simulink model "DaviAraujo_FuelHeatingModel_DashBoardOK"  (R2021a)
settings: Solver=ode5  StartTime=0.0  StopTime=inf  FixedStep=0.01  RelTol=1e-3
values from neighbouring files (symbols this model uses):
  A = 0.0003*4    (= 0.0012)    [FuelHeatingModel_WS.m]
  Densidade_Combustivel = 0.774    [FuelHeatingModel_WS.m]
  EngineTemp = 90    [FuelHeatingModel_WS.m]
  Fluxo_Injetor = 2.141967    [FuelHeatingModel_WS.m]
  h = 12000    [FuelHeatingModel_WS.m]
  Lead_MaxTemp = 80    [FuelHeatingModel_WS.m]
  LeadAcid_TotalEnergy = Voltage_LeadAcid*AmpHour_LeadAcid    (= 600)    [FuelHeatingModel_WS.m]
  Lithium_MaxTemp = 80    [FuelHeatingModel_WS.m]
  Lithium_TotalEnergy = Voltage_Lithium*AmpHour_Lithium    (= 768)    [FuelHeatingModel_WS.m]
  m = (0.4*0.79)    (= 0.316)    [FuelHeatingModel_WS.m]
  Pressure_Ethanol = (P_min:((P_max-P_min)/20):P_max).^4.92    [FuelHeatingModel_WS.m]
  PWM = 0:5:100    [FuelHeatingModel_WS.m]
  RPM_Motor = 1000    [FuelHeatingModel_WS.m]
  Setpoint_ColdStart = 120    [FuelHeatingModel_WS.m]
  Setpoint_PostStart = 90    [FuelHeatingModel_WS.m]
  Temp_Ethanol = 0:6:120    [FuelHeatingModel_WS.m]
  Ts = (Ts_min:((Ts_max-Ts_min)/20):Ts_max).^0.7    [FuelHeatingModel_WS.m]
  VolumeInterno_CommonRail = 7000    [FuelHeatingModel_WS.m]
libraries: simulink x4
(part 2 of 2)

== system DaviAraujo_FuelHeatingModel_DashBoardOK/Function-Call Subsystem/Controlador de Aquecimento Pós Partida/Transient Engine ON - Fuel Heating System/Determinação do Fluxo de Combustível ==
  Fuel Density : Inport
  Fuel Pulse Width : Inport  Port=2
  Engine Speed : Inport  Port=3
  Injector Fuel Flow : Inport  Port=4
  Divide : Product  Inputs=*/
  Duração do Ciclo (ms) : Product  Inputs=*/
  Fluxo de Combustível Normalizado (mg/ms) : Product  Inputs=**
  Min to ms : Constant  Value=60000
  Normalized Fuel Flow (mm³/ms) : Product  Inputs=*/
  Pulso de Injeção (mg/cyc) : Product  Inputs=**
  Fuel Flow mm³/ms : Outport
  wires:
  Engine Speed/1 -> Duração do Ciclo (ms)/2
  Fluxo de Combustível Normalizado (mg/ms)/1 -> Normalized Fuel Flow (mm³/ms)/1
  Duração do Ciclo (ms)/1 -> Divide/2
  Divide/1 -> Fluxo de Combustível Normalizado (mg/ms)/1
  Pulso de Injeção (mg/cyc)/1 -> Divide/1
  Injector Fuel Flow/1 -> Pulso de Injeção (mg/cyc)/2, Fluxo de Combustível Normalizado (mg/ms)/2
  Fuel Pulse Width/1 -> Pulso de Injeção (mg/cyc)/1
  Normalized Fuel Flow (mm³/ms)/1 -> Fuel Flow mm³/ms/1
  Min to ms/1 -> Duração do Ciclo (ms)/1
  Fuel Density/1 -> [Densidade_Combustivel]
  [Densidade_Combustivel] -> Normalized Fuel Flow (mm³/ms)/2

== stateflow chart DaviAraujo_FuelHeatingModel_DashBoardOK/Function-Call Subsystem/Controlador de Limitador de PWM/Timer ==
  state Power_Modulated_PWM
    entry:t_mod_cont=0;
    during:t_mod_cont=t_mod_cont+0.01;
    during:t_mod=t_mod+0.01;
  state Full_PWM
    entry:t_full_cont=0
    during:t_full_cont=t_full_cont+0.01;
    during:t_full=t_full+0.01;
  state DoorReset
    entry:t_mod_cont=0; t_mod=0;
    entry:t_full_cont=0; t_full=0;
  (default) -> Full_PWM : {t_mod=0;t_full=0;}
  Power_Modulated_PWM -> Full_PWM [order 1] : [PWM>=50]
  Full_PWM -> Power_Modulated_PWM : [PWM<50&&PWM~=0]
  DoorReset -> Full_PWM : [BCM_DoorOpen==1]
  Power_Modulated_PWM -> DoorReset [order 2] : [BCM_DoorOpen==0]
  data: PWM input; t_full_cont output; t_mod_cont output; t_full output; t_mod output; BCM_DoorOpen input

== stateflow chart DaviAraujo_FuelHeatingModel_DashBoardOK/Function-Call Subsystem/Condições de Ativação/FuSa 5/Battery Selector  ==
  note: This block meets the following requirements:
      | -Funtional Requirements 17.3 and 17.4
      | -FuSa Requirement 5
  state LeadAcid_Selected
    during:BatterySelector=1;
  state BatteriesTooHot
    during:BatterySelector=0;
  state Lithium_Selected
    during:BatterySelector=2;
  (default) -> LeadAcid_Selected
  BatteriesTooHot -> LeadAcid_Selected [order 1] : [BMS_Lead_Temp<0.6*Lead_MaxTemp]
  LeadAcid_Selected -> BatteriesTooHot [order 1] : [BMS_Lead_Temp>Lead_MaxTemp&&...
      | BMS_Lithium_Temp>Lithium_MaxTemp]
  LeadAcid_Selected -> Lithium_Selected [order 2] : [(BMS_Lead_SoC<50&&BMS_Lithium_SoC>50)...
      | ||BMS_Lead_Temp>Lead_MaxTemp]
  Lithium_Selected -> LeadAcid_Selected [order 2] : [BMS_Lithium_SoC<50]
  Lithium_Selected -> BatteriesTooHot [order 1] : [BMS_Lead_Temp>Lead_MaxTemp&&...
      | BMS_Lithium_Temp>Lithium_MaxTemp]
  BatteriesTooHot -> Lithium_Selected [order 2] : [BMS_Lithium_Temp<0.6*Lithium_MaxTemp]
  data: Lead_MaxTemp parameter; Lithium_MaxTemp parameter; BMS_Lead_SoC input; BMS_Lead_Temp input; BMS_Lithium_SoC input; BMS_Lithium_Temp input; BatterySelector output

== stateflow chart DaviAraujo_FuelHeatingModel_DashBoardOK/Function-Call Subsystem/Setpoint de Temperatura/Setpoint Adjuster ==
  note: This logic predics and prevent, any condition where the temperature setpoint is greater than the saturation temperature of the fuel for a given Comon Rail Pressure.
      | Otherwise vapor could be formed in the Comon Rail, causing problems.
  state AlowedSetpoint
    during:Real_Setpoint=DesiredSetpoint_Temp;
  state NotAllowedSetpoint
    during:Real_Setpoint=Saturation_Temp;
  (default) -> AlowedSetpoint
  NotAllowedSetpoint -> AlowedSetpoint : [DesiredSetpoint_Temp<Saturation_Temp]
  AlowedSetpoint -> NotAllowedSetpoint : [DesiredSetpoint_Temp>Saturation_Temp]
  data: DesiredSetpoint_Temp input; Saturation_Temp input; Real_Setpoint output

== stateflow chart DaviAraujo_FuelHeatingModel_DashBoardOK/Function-Call Subsystem/Condições de Ativação/Requirement 2, 14 and 15 ==
  state MalfunctionDetected
    during:DriveReady = 1;
  state KeyNotDetected
    during:Heat = 0;
    during:DriveReady = 0;
  state VehicleRunning
    during:Heat = 1;
    during:DriveReady = 2;
  state KeyDetected_ColdStart
    during:Heat = 1;
    during:DriveReady = 0;
  state KeyDetected_VehicleReady
    during:Heat = 0;
    during:DriveReady = 1;
    exit:DriveReady = 0;
  state StarterMotor_ON
    entry:count=0;
    during:count = count + 0.01;
    during:Heat = 0;
  state VehicleReadyToStart
    during:Heat = 1;
    during:DriveReady = 1;
    exit:DriveReady = 1;
  MalfunctionDetected -> KeyNotDetected [order 1] : [BCM_KeyDetector==0]
  MalfunctionDetected -> StarterMotor_ON [order 2] : [StartStopButton==1]
  KeyNotDetected -> MalfunctionDetected [order 1] : [BCM_KeyDetector==1&&Malfunction==0]
  (default) -> KeyNotDetected : {Heat = 0; DriveReady = 0;}
  VehicleRunning -> KeyNotDetected : [BCM_KeyDetector==0||StartStopButton==0]
  VehicleReadyToStart -> KeyNotDetected [order 1] : [BCM_KeyDetector==0]
  KeyNotDetected -> KeyDetected_VehicleReady [order 2] : [ECU_EngCoolant_Temp>=25 &&...
      | BCM_KeyDetector==1]
  KeyDetected_ColdStart -> KeyNotDetected [order 1] : [BCM_KeyDetector==0]
  KeyNotDetected -> KeyDetected_ColdStart [order 3] : [BCM_KeyDetector==1]
  StarterMotor_ON -> VehicleRunning : [count>=3]
  KeyDetected_VehicleReady -> StarterMotor_ON : [StartStopButton==1]
  KeyDetected_ColdStart -> VehicleReadyToStart [order 2] : [ComonRail_FuelTemp>=0.97*AdjustedSetpoint_Temp]
  VehicleReadyToStart -> StarterMotor_ON [order 2] : [StartStopButton==1]
  data: Heat output; ComonRail_FuelTemp input; AdjustedSetpoint_Temp input; count local; DriveReady output; BCM_KeyDetector input; ECU_EngCoolant_Temp input; StartStopButton input; Malfunction input
